simulink model "laneChangeNonLinCar"  (R2020a)
settings: Solver=VariableStepAuto  StartTime=0.0  StopTime=5  MaxStep=1e-3  RelTol=1e-3  EnableMultiTasking=on
values from neighbouring files (symbols this model uses):
  V = x(4)    [myobstacleVehicleModelCT.m]    (also in myobstacleVehicleModelDT.m)
undefined symbols (not defined in the file or in its folder): Ts, u0, x0, Yref
libraries: mympclib x1, sim3dlib x1, vdynlib x1
settings Model: Creator=The MathWorks, Inc.  LastModifiedBy=kohei
settings SolverCC: AlgebraicLoopSolver=LineSearch  MinimalZcImpactIntegration=on
settings DataIOCC: LimitDataPoints=on  SaveFormat=Array  SaveOutput=off  DSMLogging=off  SaveTime=off  ReturnWorkspaceOutputs=off
settings OptimizationCC: LifeSpan=inf
settings DebuggingCC: AlgebraicLoopMsg=none  UnderspecifiedInitializationDetection=Classic  MergeDetectMultiDrivingBlocksExec=none  SolverPrmCheckMsg=warning  AllowSymbolicDim=off  StateNameClashWarn=warning  SFUnexpectedBacktrackingDiag=warning  SFNoUnconditionalDefaultTransitionDiag=warning  SFExecutionAtInitializationDiag=none  ArithmeticOperatorsInVariantConditions=warning
settings HardwareCC: ProdBitPerPointer=32  ProdBitPerSizeT=32  ProdBitPerPtrDiffT=32  ProdLargestAtomicFloat=None  ProdIntDivRoundTo=Undefined  ProdEndianess=Unspecified  ProdWordSize=32  ProdHWDeviceType=32-bit Generic
settings ModelReferenceCC: PropagateSignalLabelsOutOfModel=off
settings SFSimCC: SimUseLocalCustomCode=off  CustomCodeUndefinedFunction=UseInterfaceOnly
settings RTWCC: RTWUseLocalCustomCode=off
settings CodeAppCC: StateflowObjectComments=on
settings GRTTargetCC: TargetLangStandard=C89/C90 (ANSI)
settings ConfigComp: CovMetricSettings=dw  CovHtmlReporting=on  CovSaveCumulativeToWorkspaceVar=on  CovSaveSingleToWorkspaceVar=on  CovExternalEMLEnable=off  CovSFcnEnable=off
settings SimscapeCC: SimscapeNormalizeSystem=off  SimscapeNominalValues="[{\"value\":\"10\",\"unit\":\"V\"},{\"value\":\"1\",\"unit\":\"A\"},{\"value\":\"10\",\"unit\":\"N*m\"},{\"value\":\"10\",\"unit\":\"bar\"},{\"value\":\"100\",\"unit\":\"kJ/kg\"},{\"value\":\"1\",\"unit\":\"kW\"},{\"value\":\"300\",\"unit\":\"K\"},{\"value\":\"100\",\"unit\":\"cm^3/s\"},{\"value\":\"1\",\"unit\":\"kN\"},{\"value\":\"1\",\"unit\":\"g/cm^3\"},{\"value\":\"1\",\"unit\":\"l\"},{\"value\":\"1\",\"unit\":\"cm^2\"},{\"value\":\"60\",\"unit\":\"Hz\"}]"
settings ConfigurationSet: Description=SimMechanics 2G
settings ExplorerConfigSet: InternalSimMechanicsExplorerSettings="<ExplorerConfiguration><canonicalview>default</canonicalview><AnimationSetting><BasePlaybackSpeed>1.0</BasePlaybackSpeed><PlaybackSpeedFactor>1.0</PlaybackSpeedFactor></AnimationSetting><TilePanel><TileInfo><Tiles Columns=\"1\" Count=\"1\" Rows=\"1\"><Column Left=\"2\" Weight=\"1\"/><Column Left=\"1552\"/><Row Top=\"2\" Weight=\"1\"/><Row Top=\"932\"/><Tile Height=\"1\" Width=\"1\" X=\"0\" Y=\"0\"/></Tiles></TileInfo><SceneInfo><SceneViewer><BGColor><R>0.60000002384185791</R><G>0.60000002384185791</G><B>0.60000002384185791</B></BGColor><Camera><Position><X>0.027865189060748197</X><Y>-2.5719092456962986</Y><Z>0.23157896538506753</Z></Position><Center><X>0.62659712312732463</X><Y>-0.46110119691712204</Y><Z>0.22087365386473376</Z></Center><Up><X>-0.0079438354874226333</X><Y>0.0073246425924307582</Y><Z>0.99994162084025784</Z></Up><Left>-0.24533778208815546</Left><Right>0.24533778208815546</Right><Bottom>-0.79734779727023208</Bottom><Top>0.79734779727023208</Top></Camera></SceneViewer></SceneInfo></TilePanel></ExplorerConfiguration>"

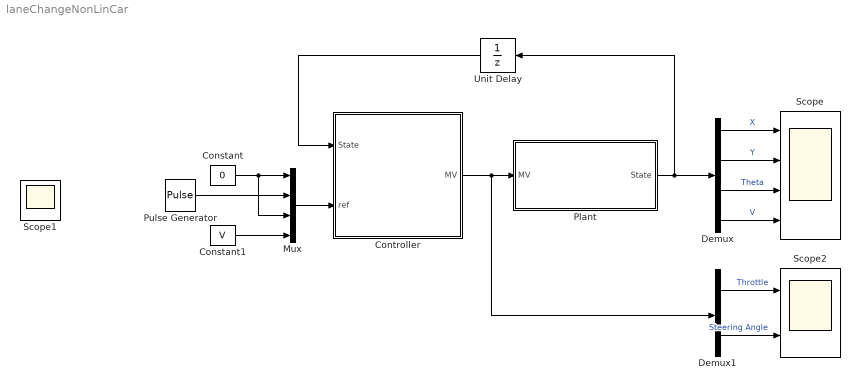
== system laneChangeNonLinCar ==
  Constant : Constant  Value=0
  Constant1 : Constant  Value=V
  Controller : Subsystem  TreatAsAtomicUnit=on
  Demux : Demux
  Demux1 : Demux  Outputs=2
  Mux : Mux
  Plant : Subsystem  TreatAsAtomicUnit=on
      mask Display: image('car.jpg')
  Pulse Generator : DiscretePulseGenerator  PulseType=Time based  Amplitude=Yref  Period=10  PulseWidth=50
  Scope : Scope  NumInputPorts=4
  Scope2 : Scope  NumInputPorts=2
  Unit Delay : UnitDelay  InitialCondition=x0  SampleTime=-1  HasFrameUpgradeWarning=on
  Scope1 : Scope
  wires:
  Demux/4 -> Scope/4  "V"
  Demux/3 -> Scope/3  "Theta"
  Demux/2 -> Scope/2  "Y"
  Demux/1 -> Scope/1  "X"
  Demux1/1 -> Scope2/1  "Throttle"
  Demux1/2 -> Scope2/2  "Steering Angle"
  Controller/1(MV) -> Plant/1(MV), Demux1/1
  Pulse Generator/1 -> Mux/2
  Mux/1 -> Controller/2(ref)
  Constant1/1 -> Mux/4
  Constant/1 -> Mux/1, Mux/3
  Plant/1(State) -> Unit Delay/1, Demux/1
  Unit Delay/1 -> Controller/1(State)

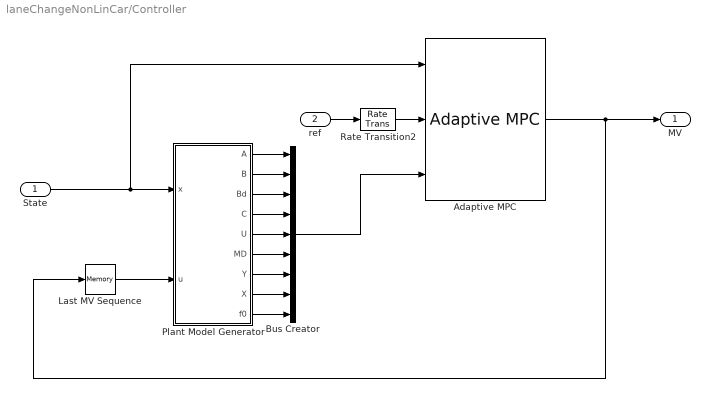
== system laneChangeNonLinCar/Controller ==
  State : Inport
  ref : Inport  Port=2
  Adaptive MPC : mympclib/Adaptive MPC  params=params  numState=4  numRef=4  numMV=2  Ts=Ts  enableDist=off  numDist=1  enableSlack=off  enableStatus=off  enableMVseq=off
      settings: SourceProductName=My MPC Library
  Bus Creator : BusCreator  Inputs=9  OutDataTypeStr=Bus: sysBus
  Last MV Sequence : Memory  InitialCondition=u0  InheritSampleTime=on
  Plant Model Generator : MATLAB Function  TreatAsAtomicUnit=on
  Rate Transition2 : RateTransition
  MV : Outport
  wires:
  Plant Model Generator/7(Y) -> Bus Creator/7
  Plant Model Generator/1(A) -> Bus Creator/1
  Plant Model Generator/8(X) -> Bus Creator/8
  Plant Model Generator/9(f0) -> Bus Creator/9
  Last MV Sequence/1 -> Plant Model Generator/2(u)
  Plant Model Generator/6(MD) -> Bus Creator/6
  Plant Model Generator/3(Bd) -> Bus Creator/3
  Plant Model Generator/2(B) -> Bus Creator/2
  Plant Model Generator/5(U) -> Bus Creator/5
  Plant Model Generator/4(C) -> Bus Creator/4
  Bus Creator/1 -> Adaptive MPC/3
  Adaptive MPC/1 -> Last MV Sequence/1, MV/1
  ref/1 -> Rate Transition2/1
  State/1 -> Adaptive MPC/1, Plant Model Generator/1(x)
  Rate Transition2/1 -> Adaptive MPC/2

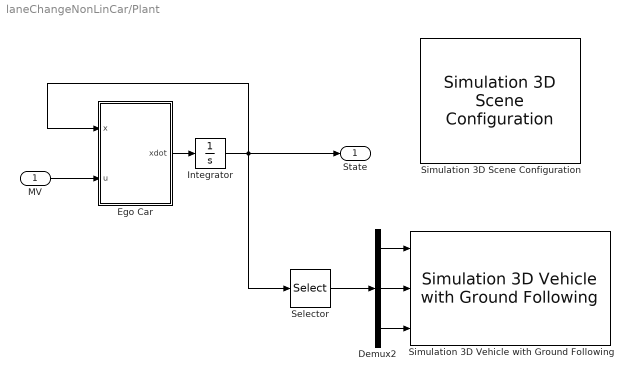
== system laneChangeNonLinCar/Plant ==
  MV : Inport
  Demux2 : Demux  Outputs=3
  Ego Car : MATLAB Function  TreatAsAtomicUnit=on  SystemSampleTime=0
  Integrator : Integrator  InitialCondition=x0
  Selector : Selector  InputPortWidth=4  IndexOptions=Index vector (dialog)  Indices=[1 2 3]  OutputSizes=1
  Simulation 3D Scene Configuration : sim3dlib/Simulation 3D Scene Configuration  Priority=0  ProjectFormat=Default Scenes  SceneDesc=Straight road  ProjectName=VehicleSimulation.exe  ScenePath=/Game/Maps/HwStrght  vehTagList={'Scene Origin';'SimulinkVehicle1'}  vehTag=SimulinkVehicle1  OpVisEn=off  Ts=.02  EnableWindow=on  sensorTag=MainCamera1  sensorId=1  sensorName=MainCamera1  mountLoc=Origin  offsetFlag=off  tmountOffset=[0, 0, 0]  rmountOffset=[0, 0, 0]  HorizontalResolution=1280  VerticalResolution=720  HorizontalFOV=60  mountPoint=[0 0 0]  mountOrientation=[0 0 0]  aMode=2  ID=1
      settings: SourceProductBaseCode=DR,VE
  Simulation 3D Vehicle with Ground Following : vdynlib/Vehicle Scenarios/Sim3D/Sim3D Vehicle/Components/Simulation 3D Vehicle with Ground Following  Priority=-1  PassVehMesh=Muscle car  VehColor=Red  InitialPos=[0, 0, 0]  InitialRot=[0, 0, 0]  ActorName=SimulinkVehicle1  SampleTime=-1  ActorType=SimulinkVehicle  ID=1  aMode=2  ActorTag=SimulinkVehicle1  CoordinateScheme=SAE
      settings: SourceProductBaseCode=VE
  State : Outport
  wires:
  MV/1 -> Ego Car/2(u)
  Integrator/1 -> State/1, Ego Car/1(x), Selector/1
  Demux2/3 -> Simulation 3D Vehicle with Ground Following/3
  Selector/1 -> Demux2/1
  Demux2/2 -> Simulation 3D Vehicle with Ground Following/2
  Demux2/1 -> Simulation 3D Vehicle with Ground Following/1
  Ego Car/1(xdot) -> Integrator/1

== matlab function laneChangeNonLinCar/Plant/Ego Car ==
  settings: updateMethod=DISCRETE  sampleTime=Ts
  data: x input; u input; xdot output
function xdot = fcn(x,u)
xdot = myobstacleVehicleModelCT(x,u);

== matlab function laneChangeNonLinCar/Controller/Plant Model Generator ==
  settings: updateMethod=DISCRETE  sampleTime=Ts
  data: x input; u input; A output; B output; Bd output; C output; U output size=[2,1]; MD output; Y output; X output size=[4,1]; f0 output; Ts parameter
function [A,B,Bd,C,U,MD,Y,X,f0] = fcn(x,u,Ts)
[A,B,Bd,C,U,MD,Y,X,f0] = myobstacleVehicleModelDT(Ts,x,u);
